simulink model "pos_state_control_simu"  (R2020b)
settings: Solver=VariableStepAuto  StartTime=0.0  StopTime=tfinal  RelTol=1e-3
values from neighbouring files (symbols this model uses):
  A = [0,1;0,-1/T]    [exp_pos_state_control.m]    (also in pos_state_control.m; pos_state_control1.m)
  B = [0;K/T]    [exp_pos_state_control.m]    (also in pos_state_control.m; pos_state_control1.m)
  C = [1,0]    [exp_pos_state_control.m]    (also in pos_state_control.m; pos_state_control1.m)
  K = 37.5    [exp_pos_state_control.m]    (also in pos_state_control.m; pos_state_control1.m)
  T = 0.107    [exp_pos_state_control.m]    (also in pos_state_control.m; pos_state_control1.m)
  theta0 = 0    [exp_pos_state_control.m]    (also in pos_state_control.m; pos_state_control1.m)
  x0 = [theta0;omega0]    [exp_pos_state_control.m]    (also in pos_state_control.m; pos_state_control1.m)
settings Model: Creator=kei55  LastModifiedBy=kei55

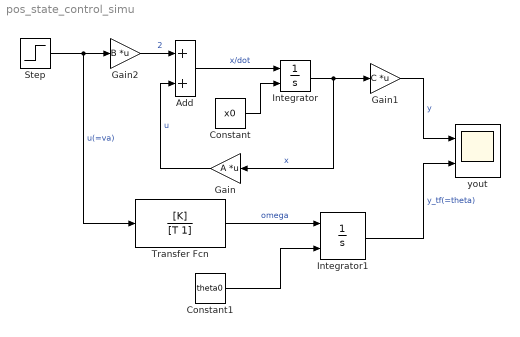
== system pos_state_control_simu ==
  Add : Sum
  Constant : Constant  Value=x0  VectorParams1D=off
  Constant1 : Constant  Value=theta0
  Gain : Gain  Gain=A  Multiplication=Matrix(K*u)
  Gain1 : Gain  Gain=C  Multiplication=Matrix(K*u)
  Gain2 : Gain  Gain=B  Multiplication=Matrix(K*u)
  Integrator : Integrator  InitialConditionSource=external
  Integrator1 : Integrator  InitialConditionSource=external
  Step : Step  SampleTime=0
  Transfer Fcn : TransferFcn  Numerator=[K]  Denominator=[T 1]
  yout : Scope  NumInputPorts=2
  wires:
  Add/1 -> Integrator/1  "x/dot"
  Integrator/1 -> Gain1/1, Gain/1  "x"
  Gain2/1 -> Add/1  "2"
  Gain/1 -> Add/2  "u"
  Gain1/1 -> yout/1  "y"
  Step/1 -> Transfer Fcn/1, Gain2/1  "u(=va)"
  Constant/1 -> Integrator/2
  Transfer Fcn/1 -> Integrator1/1  "omega"
  Constant1/1 -> Integrator1/2
  Integrator1/1 -> yout/2  "y_tf(=theta)"
